simulink model "hcc_sm_v6_circuit"  (R2024b)
settings: Solver=VariableStepAuto  StartTime=0.0  StopTime=0.2  FixedStep=1e-7  RelTol=1e-3
libraries: spsSeriesRLCBranchLib x530, spsGtoLib x144, spsDiodeLib x78, spsCurrentMeasurementLib x6, spsVoltageMeasurementLib x6, spsGroundLib x3, spsDCVoltageSourceLib x1, spsThreePhaseProgrammableVoltageSourceLib x1, spsThreePhaseTransformerTwoWindingsLib x1, spsThreePhaseSourceLib x1, spspowerguiLib x1
(part 1 of 3)
settings Model: Creator=56305  LastModifiedBy=wei13
settings SolverCC: EnableFixedStepZeroCrossing=on
settings OptimizationCC: ReuseModelBlockBuffer=off
settings RTWCC: GPUComputeCapability=3.5

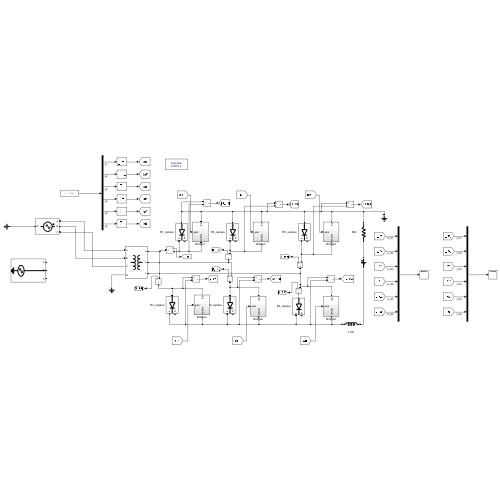
[thumbnail: Simulink's stored preview of the top-level diagram]
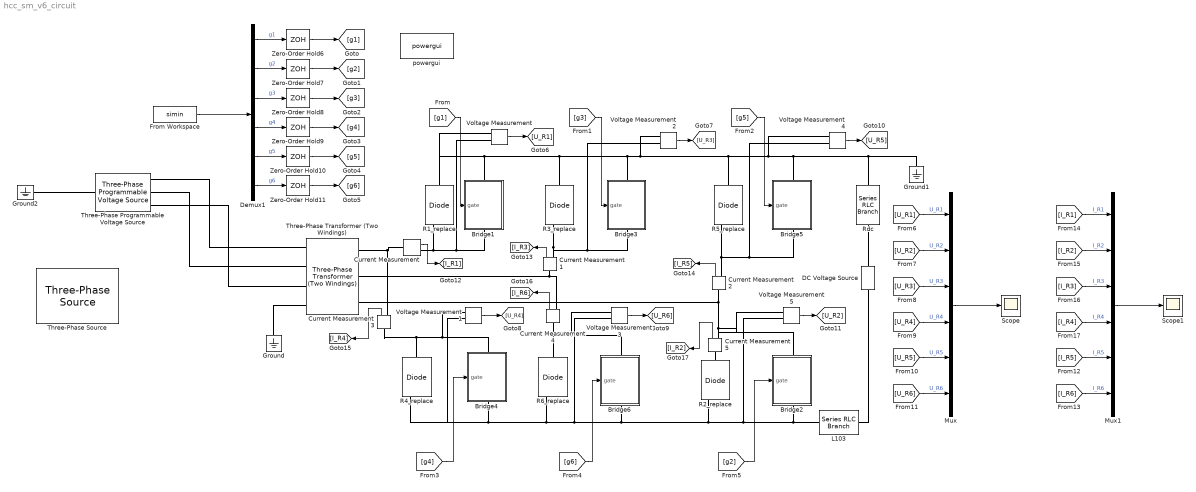
== system hcc_sm_v6_circuit ==
  Bridge1 : Subsystem
      settings: PortSchema="{\"entries\":[{\"content\":{\"sides\":[{\"content\":{\"connectorIds\":[\"In1\"]},\"type\":\"ConnectorPlacement.EquallySpacedRectSide\",\"uuid\":\"41aa3e2a-70f0-4b77-aa16-68e99ec54bcf\"},{\"content\":{\"side\":\"RIGHT\"},\"type\":\"ConnectorPlacement.EquallySpacedRectSide\",\"uuid\":\"96eb3ac2-20ab-4313-b955-709dae12ba5a\"},{\"content\":{\"connectorIds\":[\"LConn1\"],\"side\":\"TOP\"},\"type\":\"ConnectorPlacement.EquallySpacedRectSide\",\"uuid\":\"75cf1ed1-d1d6-43fb-a0f7-eae0627f950f\"},{\"content\":{\"connectorIds\":[\"RConn1\"],\"side\":\"BOTTOM\"},\"type\":\"ConnectorPlacement.EquallySpacedRectSide\",\"uuid\":\"e3d24c16-695e-4958-a9e5-c1041aebacaf\"}]},\"type\":\"ConnectorPlacement.EquallySpacedConnector\",\"uuid\":\"cea135f8-b684-4f22-bc6f-773380cf8880\"}],\"packageUris\":[\"http://schema.mathworks.com/mf0/Connector/R2020b\"],\"version\":\"1.0\"}"
  Bridge2 : Subsystem
      settings: PortSchema="{\"entries\":[{\"content\":{\"sides\":[{\"content\":{\"connectorIds\":[\"In1\"]},\"type\":\"ConnectorPlacement.EquallySpacedRectSide\",\"uuid\":\"41aa3e2a-70f0-4b77-aa16-68e99ec54bcf\"},{\"content\":{\"side\":\"RIGHT\"},\"type\":\"ConnectorPlacement.EquallySpacedRectSide\",\"uuid\":\"96eb3ac2-20ab-4313-b955-709dae12ba5a\"},{\"content\":{\"connectorIds\":[\"LConn1\"],\"side\":\"TOP\"},\"type\":\"ConnectorPlacement.EquallySpacedRectSide\",\"uuid\":\"75cf1ed1-d1d6-43fb-a0f7-eae0627f950f\"},{\"content\":{\"connectorIds\":[\"RConn1\"],\"side\":\"BOTTOM\"},\"type\":\"ConnectorPlacement.EquallySpacedRectSide\",\"uuid\":\"e3d24c16-695e-4958-a9e5-c1041aebacaf\"}]},\"type\":\"ConnectorPlacement.EquallySpacedConnector\",\"uuid\":\"cea135f8-b684-4f22-bc6f-773380cf8880\"}],\"packageUris\":[\"http://schema.mathworks.com/mf0/Connector/R2020b\"],\"version\":\"1.0\"}"
  Bridge3 : Subsystem
      settings: PortSchema="{\"entries\":[{\"content\":{\"sides\":[{\"content\":{\"connectorIds\":[\"In1\"]},\"type\":\"ConnectorPlacement.EquallySpacedRectSide\",\"uuid\":\"41aa3e2a-70f0-4b77-aa16-68e99ec54bcf\"},{\"content\":{\"side\":\"RIGHT\"},\"type\":\"ConnectorPlacement.EquallySpacedRectSide\",\"uuid\":\"96eb3ac2-20ab-4313-b955-709dae12ba5a\"},{\"content\":{\"connectorIds\":[\"LConn1\"],\"side\":\"TOP\"},\"type\":\"ConnectorPlacement.EquallySpacedRectSide\",\"uuid\":\"75cf1ed1-d1d6-43fb-a0f7-eae0627f950f\"},{\"content\":{\"connectorIds\":[\"RConn1\"],\"side\":\"BOTTOM\"},\"type\":\"ConnectorPlacement.EquallySpacedRectSide\",\"uuid\":\"e3d24c16-695e-4958-a9e5-c1041aebacaf\"}]},\"type\":\"ConnectorPlacement.EquallySpacedConnector\",\"uuid\":\"cea135f8-b684-4f22-bc6f-773380cf8880\"}],\"packageUris\":[\"http://schema.mathworks.com/mf0/Connector/R2020b\"],\"version\":\"1.0\"}"
  Bridge4 : Subsystem
      settings: PortSchema="{\"entries\":[{\"content\":{\"sides\":[{\"content\":{\"connectorIds\":[\"In1\"]},\"type\":\"ConnectorPlacement.EquallySpacedRectSide\",\"uuid\":\"41aa3e2a-70f0-4b77-aa16-68e99ec54bcf\"},{\"content\":{\"side\":\"RIGHT\"},\"type\":\"ConnectorPlacement.EquallySpacedRectSide\",\"uuid\":\"96eb3ac2-20ab-4313-b955-709dae12ba5a\"},{\"content\":{\"connectorIds\":[\"LConn1\"],\"side\":\"TOP\"},\"type\":\"ConnectorPlacement.EquallySpacedRectSide\",\"uuid\":\"75cf1ed1-d1d6-43fb-a0f7-eae0627f950f\"},{\"content\":{\"connectorIds\":[\"RConn1\"],\"side\":\"BOTTOM\"},\"type\":\"ConnectorPlacement.EquallySpacedRectSide\",\"uuid\":\"e3d24c16-695e-4958-a9e5-c1041aebacaf\"}]},\"type\":\"ConnectorPlacement.EquallySpacedConnector\",\"uuid\":\"cea135f8-b684-4f22-bc6f-773380cf8880\"}],\"packageUris\":[\"http://schema.mathworks.com/mf0/Connector/R2020b\"],\"version\":\"1.0\"}"
  Bridge5 : Subsystem
      settings: PortSchema="{\"entries\":[{\"content\":{\"sides\":[{\"content\":{\"connectorIds\":[\"In1\"]},\"type\":\"ConnectorPlacement.EquallySpacedRectSide\",\"uuid\":\"41aa3e2a-70f0-4b77-aa16-68e99ec54bcf\"},{\"content\":{\"side\":\"RIGHT\"},\"type\":\"ConnectorPlacement.EquallySpacedRectSide\",\"uuid\":\"96eb3ac2-20ab-4313-b955-709dae12ba5a\"},{\"content\":{\"connectorIds\":[\"LConn1\"],\"side\":\"TOP\"},\"type\":\"ConnectorPlacement.EquallySpacedRectSide\",\"uuid\":\"75cf1ed1-d1d6-43fb-a0f7-eae0627f950f\"},{\"content\":{\"connectorIds\":[\"RConn1\"],\"side\":\"BOTTOM\"},\"type\":\"ConnectorPlacement.EquallySpacedRectSide\",\"uuid\":\"e3d24c16-695e-4958-a9e5-c1041aebacaf\"}]},\"type\":\"ConnectorPlacement.EquallySpacedConnector\",\"uuid\":\"cea135f8-b684-4f22-bc6f-773380cf8880\"}],\"packageUris\":[\"http://schema.mathworks.com/mf0/Connector/R2020b\"],\"version\":\"1.0\"}"
  Bridge6 : Subsystem
      settings: PortSchema="{\"entries\":[{\"content\":{\"sides\":[{\"content\":{\"connectorIds\":[\"In1\"]},\"type\":\"ConnectorPlacement.EquallySpacedRectSide\",\"uuid\":\"41aa3e2a-70f0-4b77-aa16-68e99ec54bcf\"},{\"content\":{\"side\":\"RIGHT\"},\"type\":\"ConnectorPlacement.EquallySpacedRectSide\",\"uuid\":\"96eb3ac2-20ab-4313-b955-709dae12ba5a\"},{\"content\":{\"connectorIds\":[\"LConn1\"],\"side\":\"TOP\"},\"type\":\"ConnectorPlacement.EquallySpacedRectSide\",\"uuid\":\"75cf1ed1-d1d6-43fb-a0f7-eae0627f950f\"},{\"content\":{\"connectorIds\":[\"RConn1\"],\"side\":\"BOTTOM\"},\"type\":\"ConnectorPlacement.EquallySpacedRectSide\",\"uuid\":\"e3d24c16-695e-4958-a9e5-c1041aebacaf\"}]},\"type\":\"ConnectorPlacement.EquallySpacedConnector\",\"uuid\":\"cea135f8-b684-4f22-bc6f-773380cf8880\"}],\"packageUris\":[\"http://schema.mathworks.com/mf0/Connector/R2020b\"],\"version\":\"1.0\"}"
  Current Measurement{,1..5} (6 alike) : spsCurrentMeasurementLib/Current Measurement  PhasorSimulation=off  OutputType=Complex  PSBequivalent=0
  DC Voltage Source : spsDCVoltageSourceLib/DC Voltage Source  Amplitude=57000  Measurements=None
  Demux1 : Demux  Outputs=6
  From Workspace : FromWorkspace  VariableName=simin  SampleTime=0.0001  Interpolate=off  OutputAfterFinalValue=Holding final value
  Ground : spsGroundLib/Ground  LConnTagsString=a
  Ground1 : spsGroundLib/Ground  LConnTagsString=a
  Ground2 : spsGroundLib/Ground  LConnTagsString=a
  L103 : spsSeriesRLCBranchLib/Series RLC Branch  LConnTagsString=__new0  RConnTagsString=__new0  BranchType=L  Resistance=36  Inductance=120*1e-03  SetiL0=off  InitialCurrent=0  Capacitance=2.62e-06  Setx0=off  InitialVoltage=0  Measurements=None
  Mux : Mux  Inputs=6
  Mux1 : Mux  Inputs=6
  R1_replace : spsDiodeLib/Diode  Ron=3.2041  Lon=0  Vf=119772.7273  IC=0  UseSnubber=0  Rs=1e6  Cs=0  Measurements=on
  R2_replace : spsDiodeLib/Diode  Ron=3.2041  Lon=0  Vf=119772.7273  IC=0  UseSnubber=0  Rs=1e6  Cs=0  Measurements=on
  R3_replace : spsDiodeLib/Diode  Ron=3.2041  Lon=0  Vf=119772.7273  IC=0  UseSnubber=0  Rs=1e6  Cs=0  Measurements=on
  R4_replace : spsDiodeLib/Diode  Ron=3.2041  Lon=0  Vf=119772.7273  IC=0  UseSnubber=0  Rs=1e6  Cs=0  Measurements=on
  R5_replace : spsDiodeLib/Diode  Ron=3.2041  Lon=0  Vf=119772.7273  IC=0  UseSnubber=0  Rs=1e6  Cs=0  Measurements=on
  R6_replace : spsDiodeLib/Diode  Ron=3.2041  Lon=0  Vf=119772.7273  IC=0  UseSnubber=0  Rs=1e6  Cs=0  Measurements=on
  Rdc : spsSeriesRLCBranchLib/Series RLC Branch  LConnTagsString=__new0  RConnTagsString=__new0  BranchType=R  Resistance=1  Inductance=120e-03  SetiL0=off  InitialCurrent=0  Capacitance=2.62e-06  Setx0=off  InitialVoltage=0  Measurements=None
  Scope : Scope
  Scope1 : Scope
  Three-Phase Programmable Voltage Source : spsThreePhaseProgrammableVoltageSourceLib/Three-Phase Programmable Voltage Source  PositiveSequence="[345e3  0 50]"  VariationEntity=Amplitude  VariationType=Table of time-amplitude pairs  VariationTypeAlt=Step  VariationStep=0.5  VariationRate=1000  VariationMagnitude=0.3  VariationFrequency=2  VariationTiming=[0 1]  VariationPhaseA=off  Amplitudes=[0.000000 0.002000 0.004000 0.006000 0.008000 0.010000 0.012000 0.014000 0.016000 0.018000 0.020000 0.022000 0.024000 0.026000 0.028000 0.030000 0.032000 0.034000 0.036000 0.038000 0.040000 0.042000 0.044000 0.046000 0.048000 0.050000 0.052000 0.054000 0.056000 0.058000 0.060000 0.062000 0.064000 0.066000 0.068000 0.070000 0.072000 0.074000 0.076000 0.078000 0.080000 0.082000 0.084000 0.086000 0.088000 0.090000 0.092000 0.094000 0.096000 0.098000 0.100000 0.102000 0.104000 0.106000 0.108000 0.110000 0.112000 0.114000 0.116000 0.118000 0.120000 0.122000 0.124000 0.126000 0.128000 0.130000 0.132000 0.134000 0.136000 0.138000 0.140000 0.142000 0.144000 0.146000 0.148000 0.150000 0.152000 0.154000 0.156000 0.158000 0.160000 0.162000 0.164000 0.166000 0.168000 0.170000 0.172000 0.174000 0.176000 0.178000 0.180000 0.182000 0.184000 0.186000 0.188000 0.190000 0.192000 0.194000 0.196000 0.198000 0.200000 0.202000 0.204000 0.206000 0.208000 0.210000 0.212000 0.214000 0.216000 0.218000 0.220000 0.222000 0.224000 0.226000 0.228000 0.230000 0.232000 0.234000 0.236000 0.238000 0.240000 0.242000 0.244000 0.246000 0.248000 0.250000 0.252000 0.254000 0.256000 0.258000 0.260000 0.262000 0.264000 0.266000 0.268000 0.270000 0.272000 0.274000 0.276000 0.278000 0.280000 0.282000 0.284000 0.286000 0.288000 0.290000 0.292000 0.294000 0.296000 0.298000 0.300000 0.302000 0.304000 0.306000 0.308000 0.310000 0.312000 0.314000 0.316000 0.318000 0.320000 0.322000 0.324000 0.326000 0.328000 0.330000 0.332000 0.334000 0.336000 0.338000 0.340000 0.342000 0.344000 0.346000 0.348000 0.350000 0.352000 0.354000 0.356000 0.358000 0.360000 0.362000 0.364000 0.366000 0.368000 0.370000 0.372000 0.374000 0.376000 0.378000 0.380000 0.382000 0.384000 0.386000 0.388000 0.390000 0.392000 0.394000 0.396000 0.398000 0.400000 0.402000 0.404000 0.406000 0.408000 0.410000 0.412000 0.414000 0.416000 0.418000 0.420000 0.422000 0.424000 0.426000 0.428000 0.430000 0.432000 0.434000 0.436000 0.438000 0.440000 0.442000 0.444000 0.446000 0.448000 0.450000 0.452000 0.454000 0.456000 0.458000 0.460000 0.462000 0.464000 0.466000 0.468000 0.470000 0.472000 0.474000 0.476000 0.478000 0.480000 0.482000 0.484000 0.486000 0.488000 0.490000 0.492000 0.494000 0.496000 0.498000 0.500000 0.502000 0.504000 0.506000 0.508000 0.510000 0.512000 0.514000 0.516000 0.518000 0.520000 0.522000 0.524000 0.526000 0.528000 0.530000 0.532000 0.534000 0.536000 0.538000 0.540000 0.542000 0.544000 0.546000 0.548000 0.550000 0.552000 0.554000 0.556000 0.558000 0.560000 0.562000 0.564000 0.566000 0.568000 0.570000 0.572000 0.574000 0.576000 0.578000 0.580000 0.582000 0.584000 0.586000 0.588000 0.590000 0.592000 0.594000 0.596000 0.598000 0.600000 0.602000 0.604000 0.606000 0.608000 0.610000 0.612000 0.614000 0.616000 0.618000 0.620000 0.622000 0.624000 0.626000 0.628000 0.630000 0.632000 0.634000 0.636000 0.638000 0.640000 0.642000 0.644000 0.646000 0.648000 0.650000 0.652000 0.654000 0.656000 0.658000 0.660000 0.662000 0.664000 0.666000 0.668000 0.670000 0.672000 0.674000 0.676000 0.678000 0.680000 0.682000 0.684000 0.686000 0.688000 0.690000 0.692000 0.694000 0.696000 0.698000 0.700000 0.702000 0.704000 0.706000 0.708000 0.710000 0.712000 0.714000 0.716000 0.718000 0.720000 0.722000 0.724000 0.726000 0.728000 0.730000 0.732000 0.734000 0.736000 0.738000 0.740000 0.742000 0.744000 0.746000 0.748000 0.750000 0.752000 0.754000 0.756000 0.758000 0.760000 0.762000 0.764000 0.766000 0.768000 0.770000 0.772000 0.774000 0.776000 0.778000 0.780000 0.782000 0.784000 0.786000 0.788000 0.790000 0.792000 0.794000 0.796000 0.798000 0.800000 0.802000 0.804000 0.806000 0.808000 0.810000 0.812000 0.814000 0.816000 0.818000 0.820000 0.822000 0.824000 0.826000 0.828000 0.830000 0.832000 0.834000 0.836000 0.838000 0.840000 0.842000 0.844000 0.846000 0.848000 0.850000 0.852000 0.854000 0.856000 0.858000 0.860000 0.862000 0.864000 0.866000 0.868000 0.870000 0.872000 0.874000 0.876000 0.878000 0.880000 0.882000 0.884000 0.886000 ...(+513 chars) ]  TimeValues=[0.000000 0.000100 0.000200 0.000300 0.000400 0.000500 0.000600 0.000700 0.000800 0.000900 0.001000 0.001100 0.001200 0.001300 0.001400 0.001500 0.001600 0.001700 0.001800 0.001900 0.002000 0.002100 0.002200 0.002300 0.002400 0.002500 0.002600 0.002700 0.002800 0.002900 0.003000 0.003100 0.003200 0.003300 0.003400 0.003500 0.003600 0.003700 0.003800 0.003900 0.004000 0.004100 0.004200 0.004300 0.004400 0.004500 0.004600 0.004700 0.004800 0.004900 0.005000 0.005100 0.005200 0.005300 0.005400 0.005500 0.005600 0.005700 0.005800 0.005900 0.006000 0.006100 0.006200 0.006300 0.006400 0.006500 0.006600 0.006700 0.006800 0.006900 0.007000 0.007100 0.007200 0.007300 0.007400 0.007500 0.007600 0.007700 0.007800 0.007900 0.008000 0.008100 0.008200 0.008300 0.008400 0.008500 0.008600 0.008700 0.008800 0.008900 0.009000 0.009100 0.009200 0.009300 0.009400 0.009500 0.009600 0.009700 0.009800 0.009900 0.010000 0.010100 0.010200 0.010300 0.010400 0.010500 0.010600 0.010700 0.010800 0.010900 0.011000 0.011100 0.011200 0.011300 0.011400 0.011500 0.011600 0.011700 0.011800 0.011900 0.012000 0.012100 0.012200 0.012300 0.012400 0.012500 0.012600 0.012700 0.012800 0.012900 0.013000 0.013100 0.013200 0.013300 0.013400 0.013500 0.013600 0.013700 0.013800 0.013900 0.014000 0.014100 0.014200 0.014300 0.014400 0.014500 0.014600 0.014700 0.014800 0.014900 0.015000 0.015100 0.015200 0.015300 0.015400 0.015500 0.015600 0.015700 0.015800 0.015900 0.016000 0.016100 0.016200 0.016300 0.016400 0.016500 0.016600 0.016700 0.016800 0.016900 0.017000 0.017100 0.017200 0.017300 0.017400 0.017500 0.017600 0.017700 0.017800 0.017900 0.018000 0.018100 0.018200 0.018300 0.018400 0.018500 0.018600 0.018700 0.018800 0.018900 0.019000 0.019100 0.019200 0.019300 0.019400 0.019500 0.019600 0.019700 0.019800 0.019900 0.020000 0.020100 0.020200 0.020300 0.020400 0.020500 0.020600 0.020700 0.020800 0.020900 0.021000 0.021100 0.021200 0.021300 0.021400 0.021500 0.021600 0.021700 0.021800 0.021900 0.022000 0.022100 0.022200 0.022300 0.022400 0.022500 0.022600 0.022700 0.022800 0.022900 0.023000 0.023100 0.023200 0.023300 0.023400 0.023500 0.023600 0.023700 0.023800 0.023900 0.024000 0.024100 0.024200 0.024300 0.024400 0.024500 0.024600 0.024700 0.024800 0.024900 0.025000 0.025100 0.025200 0.025300 0.025400 0.025500 0.025600 0.025700 0.025800 0.025900 0.026000 0.026100 0.026200 0.026300 0.026400 0.026500 0.026600 0.026700 0.026800 0.026900 0.027000 0.027100 0.027200 0.027300 0.027400 0.027500 0.027600 0.027700 0.027800 0.027900 0.028000 0.028100 0.028200 0.028300 0.028400 0.028500 0.028600 0.028700 0.028800 0.028900 0.029000 0.029100 0.029200 0.029300 0.029400 0.029500 0.029600 0.029700 0.029800 0.029900 0.030000 0.030100 0.030200 0.030300 0.030400 0.030500 0.030600 0.030700 0.030800 0.030900 0.031000 0.031100 0.031200 0.031300 0.031400 0.031500 0.031600 0.031700 0.031800 0.031900 0.032000 0.032100 0.032200 0.032300 0.032400 0.032500 0.032600 0.032700 0.032800 0.032900 0.033000 0.033100 0.033200 0.033300 0.033400 0.033500 0.033600 0.033700 0.033800 0.033900 0.034000 0.034100 0.034200 0.034300 0.034400 0.034500 0.034600 0.034700 0.034800 0.034900 0.035000 0.035100 0.035200 0.035300 0.035400 0.035500 0.035600 0.035700 0.035800 0.035900 0.036000 0.036100 0.036200 0.036300 0.036400 0.036500 0.036600 0.036700 0.036800 0.036900 0.037000 0.037100 0.037200 0.037300 0.037400 0.037500 0.037600 0.037700 0.037800 0.037900 0.038000 0.038100 0.038200 0.038300 0.038400 0.038500 0.038600 0.038700 0.038800 0.038900 0.039000 0.039100 0.039200 0.039300 0.039400 0.039500 0.039600 0.039700 0.039800 0.039900 0.040000 0.040100 0.040200 0.040300 0.040400 0.040500 0.040600 0.040700 0.040800 0.040900 0.041000 0.041100 0.041200 0.041300 0.041400 0.041500 0.041600 0.041700 0.041800 0.041900 0.042000 0.042100 0.042200 0.042300 0.042400 0.042500 0.042600 0.042700 0.042800 0.042900 0.043000 0.043100 0.043200 0.043300 0.043400 0.043500 0.043600 0.043700 0.043800 0.043900 0.044000 0.044100 0.044200 0.044300 ...(+513 chars) ]  HarmonicGeneration=off  HarmonicA=[3 0.2 -25 0]  HarmonicB=[2 0.15 35 2]  Timing="[0.05  3]"  BusType=swing  Pref=0  Qref=0  Qmin=-inf  Qmax=inf
  Three-Phase Transformer (Two Windings) : spsThreePhaseTransformerTwoWindingsLib/Three-Phase Transformer (Two Windings)  Winding1Connection=Yn  Winding2Connection=Y  CoreType=Three single-phase transformers  SetSaturation=off  Hysteresis=off  DataFile='hysteresis'  SetInitialFlux=off  Measurements=None  UNITS=pu  NominalPower=[ 215.4e6 , 50 ]  Winding1=[ 345e3 , 0.002 , 0.08 ]  Winding2=[ 50.8e3 , 0.002 , 0.08 ]  Rm=500  Lm=500  L0=0.5  Saturation=[ 0,0 ; 0.0024,1.2 ; 1.0,1.52 ]  InitialFluxes=[ 0.8 , -0.8 , 0.7 ]  BreakLoop=off  DiscreteSolver=Trapezoidal iterative  DataType=off  TransfoNumber=1
  Three-Phase Source : spsThreePhaseSourceLib/Three-Phase Source  InternalConnection=Yg  VoltagePhases=off  Voltage=345e3  PhaseAngle=0  Voltage_phases=[25e3 25e3 25e3]/sqrt(3)  PhaseAngles_phases=[0 -120 +120]  Frequency=50  NonIdealSource=off  SpecifyImpedance=off  Resistance=0  Inductance=0  ShortCircuitLevel=100e6  BaseVoltage=25e3  XRratio=7  BusType=swing  Pref=10e3  Qref=0  Prefabc=[10e3, 10e3, 10e3]  Qrefabc=[0, 0, 0]  Qmin=-inf  Qmax=inf
  Voltage Measurement{,1..5} (6 alike) : spsVoltageMeasurementLib/Voltage Measurement  PhasorSimulation=off  OutputType=Complex  PSBequivalent=0
  Zero-Order Hold{6..11} (6 alike) : ZeroOrderHold  SampleTime=1e-4
  powergui : spspowerguiLib/powergui  Priority=1  SimulationMode=Discrete  SampleTime=1e-4  frequency=60  Iterations=50  frequencyindice=50  Pbase=100e6  ErrMax=1e-4  UnitsV=kV  UnitsW=MW  buscounter=0  FunctionMessages=off  echomessages=off  EnableUseOfTLC=off  CurrentSourceSwitches=off  DisableSnubberDevices=off  DisableRonSwitches=off  DisableVfSwitches=off  DisplayEquations=off  AutomaticDiscreteSolvers=off  SolverType=Tustin/Backward Euler (TBE)  Interpol=off  ExternalGateDelay=off  methode=off  Ts=100  x0status=blocks  SPID=on  SwTol=0  HookPort=off  NonlinearTolerance=1e-4  nMaxIteration=1000  ContinueOnMaxIteration=off  RestoreLinks=warning  ResistiveCurrentMeasurement=off  Frange=[0:2:500]  Ylog=off  Xlog=on  ShowGrid=off  save=off  variable=ZData  structure=0  ZoomFFT=off  StartTime=0.0  cycles=1  DisplayStyle=1  fundamental=60  FreqAxis=off  MaxFrequency=1000  frequencyindicesteady=1  RmsSteady=1  display=off
  wires:
  From Workspace/1 -> Demux1/1
  [g1] -> Bridge1/1(gate)
  [g3] -> Bridge3/1(gate)
  [g5] -> Bridge5/1(gate)
  [g4] -> Bridge4/1(gate)
  [g6] -> Bridge6/1(gate)
  [g2] -> Bridge2/1(gate)
  Voltage Measurement/1 -> [U_R1]
  Voltage Measurement2/1 -> [U_R3]
  Voltage Measurement1/1 -> [U_R4]
  Voltage Measurement3/1 -> [U_R6]
  Voltage Measurement4/1 -> [U_R5]
  Voltage Measurement5/1 -> [U_R2]
  [U_R1] -> Mux/1  "U_R1"
  [U_R2] -> Mux/2  "U_R2"
  [U_R3] -> Mux/3  "U_R3"
  [U_R4] -> Mux/4  "U_R4"
  [U_R5] -> Mux/5  "U_R5"
  [U_R6] -> Mux/6  "U_R6"
  Mux/1 -> Scope/1
  Demux1/2 -> Zero-Order Hold7/1  "g2"
  Demux1/1 -> Zero-Order Hold6/1  "g1"
  Demux1/3 -> Zero-Order Hold8/1  "g3"
  Demux1/4 -> Zero-Order Hold9/1  "g4"
  Demux1/5 -> Zero-Order Hold10/1  "g5"
  Demux1/6 -> Zero-Order Hold11/1  "g6"
  Zero-Order Hold6/1 -> [g1]
  Zero-Order Hold7/1 -> [g2]
  Zero-Order Hold8/1 -> [g3]
  Zero-Order Hold9/1 -> [g4]
  Zero-Order Hold10/1 -> [g5]
  Zero-Order Hold11/1 -> [g6]
  Current Measurement/1 -> [I_R1]
  Current Measurement1/1 -> [I_R3]
  Current Measurement2/1 -> [I_R5]
  Current Measurement3/1 -> [I_R4]
  Current Measurement4/1 -> [I_R6]
  Current Measurement5/1 -> [I_R2]
  Mux1/1 -> Scope1/1
  [I_R4] -> Mux1/4  "I_R4"
  [I_R5] -> Mux1/5  "I_R5"
  [I_R3] -> Mux1/3  "I_R3"
  [I_R2] -> Mux1/2  "I_R2"
  [I_R1] -> Mux1/1  "I_R1"
  [I_R6] -> Mux1/6  "I_R6"
  connections:
  Three-Phase Transformer (Two Windings)/LConn4 -- Ground/LConn1
  R4_replace/LConn1 -- Current Measurement3/LConn1 -- Bridge4/LConn1 -- Voltage Measurement1/LConn1
  R3_replace/RConn1 -- Bridge3/RConn1 -- Voltage Measurement2/LConn2 -- Current Measurement1/RConn1
  Three-Phase Transformer (Two Windings)/RConn3 -- Bridge2/LConn1 -- Voltage Measurement5/LConn1 -- Current Measurement5/RConn1 -- Current Measurement2/LConn1
  L103/LConn1 -- Bridge2/RConn1 -- Voltage Measurement5/LConn2 -- R2_replace/RConn1 -- Bridge6/RConn1 -- Voltage Measurement3/LConn2 -- R6_replace/RConn1 -- Bridge4/RConn1 -- Voltage Measurement1/LConn2 -- R4_replace/RConn1
  DC Voltage Source/RConn1 -- Rdc/RConn1
  Voltage Measurement/LConn1 -- R1_replace/LConn1 -- Bridge1/LConn1 -- R3_replace/LConn1 -- Bridge3/LConn1 -- Voltage Measurement2/LConn1 -- R5_replace/LConn1 -- Voltage Measurement4/LConn1 -- Bridge5/LConn1 -- Rdc/LConn1 -- Ground1/LConn1
  L103/RConn1 -- DC Voltage Source/LConn1
  Ground2/LConn1 -- Three-Phase Programmable Voltage Source/LConn1
  Three-Phase Transformer (Two Windings)/LConn3 -- Three-Phase Programmable Voltage Source/RConn3
  Three-Phase Programmable Voltage Source/RConn2 -- Three-Phase Transformer (Two Windings)/LConn2
  Three-Phase Transformer (Two Windings)/LConn1 -- Three-Phase Programmable Voltage Source/RConn1
  R1_replace/RConn1 -- Bridge1/RConn1 -- Voltage Measurement/LConn2 -- Current Measurement/RConn1
  Three-Phase Transformer (Two Windings)/RConn2 -- Current Measurement4/RConn1 -- Current Measurement1/LConn1
  Bridge5/RConn1 -- Voltage Measurement4/LConn2 -- Current Measurement2/RConn1 -- R5_replace/RConn1
  Three-Phase Transformer (Two Windings)/RConn1 -- Current Measurement3/RConn1 -- Current Measurement/LConn1
  R6_replace/LConn1 -- Current Measurement4/LConn1 -- Bridge6/LConn1 -- Voltage Measurement3/LConn1
  Current Measurement5/LConn1 -- R2_replace/LConn1

== system hcc_sm_v6_circuit/Bridge1 ==
  gate : Inport
  Segment1 : Subsystem
  Segment2 : Subsystem
  Segment3 : Subsystem
  Segment4 : Subsystem
  top : PMIOPort  Side=Left
  bottom : PMIOPort  Port=2  Side=Right
  wires:
  gate/1 -> Segment2/1(gate), Segment4/1(gate), Segment3/1(gate), Segment1/1(gate)
  connections:
  Segment2/LConn1 -- Segment1/RConn1
  Segment3/LConn1 -- Segment2/RConn1
  Segment4/LConn1 -- Segment3/RConn1
  Segment1/LConn1 -- top/RConn1
  Segment4/RConn1 -- bottom/RConn1

== system hcc_sm_v6_circuit/Bridge2 ==
  gate : Inport
  Segment1 : Subsystem
  Segment2 : Subsystem
  Segment3 : Subsystem
  Segment4 : Subsystem
  top : PMIOPort  Side=Left
  bottom : PMIOPort  Port=2  Side=Right
  wires:
  gate/1 -> Segment1/1(gate), Segment3/1(gate), Segment4/1(gate), Segment2/1(gate)
  connections:
  Segment4/RConn1 -- bottom/RConn1
  Segment1/LConn1 -- top/RConn1
  Segment4/LConn1 -- Segment3/RConn1
  Segment3/LConn1 -- Segment2/RConn1
  Segment2/LConn1 -- Segment1/RConn1

== system hcc_sm_v6_circuit/Bridge3 ==
  gate : Inport
  Segment1 : Subsystem
  Segment2 : Subsystem
  Segment3 : Subsystem
  Segment4 : Subsystem
  top : PMIOPort  Side=Left
  bottom : PMIOPort  Port=2  Side=Right
  wires:
  gate/1 -> Segment2/1(gate), Segment4/1(gate), Segment3/1(gate), Segment1/1(gate)
  connections:
  Segment2/LConn1 -- Segment1/RConn1
  Segment3/LConn1 -- Segment2/RConn1
  Segment4/LConn1 -- Segment3/RConn1
  Segment1/LConn1 -- top/RConn1
  Segment4/RConn1 -- bottom/RConn1

== system hcc_sm_v6_circuit/Bridge4 ==
  gate : Inport
  Segment1 : Subsystem
  Segment2 : Subsystem
  Segment3 : Subsystem
  Segment4 : Subsystem
  top : PMIOPort  Side=Left
  bottom : PMIOPort  Port=2  Side=Right
  wires:
  gate/1 -> Segment1/1(gate), Segment3/1(gate), Segment4/1(gate), Segment2/1(gate)
  connections:
  Segment4/RConn1 -- bottom/RConn1
  Segment1/LConn1 -- top/RConn1
  Segment4/LConn1 -- Segment3/RConn1
  Segment3/LConn1 -- Segment2/RConn1
  Segment2/LConn1 -- Segment1/RConn1

== system hcc_sm_v6_circuit/Bridge5 ==
  gate : Inport
  Segment1 : Subsystem
  Segment2 : Subsystem
  Segment3 : Subsystem
  Segment4 : Subsystem
  top : PMIOPort  Side=Left
  bottom : PMIOPort  Port=2  Side=Right
  wires:
  gate/1 -> Segment2/1(gate), Segment4/1(gate), Segment3/1(gate), Segment1/1(gate)
  connections:
  Segment2/LConn1 -- Segment1/RConn1
  Segment3/LConn1 -- Segment2/RConn1
  Segment4/LConn1 -- Segment3/RConn1
  Segment1/LConn1 -- top/RConn1
  Segment4/RConn1 -- bottom/RConn1

== system hcc_sm_v6_circuit/Bridge6 ==
  gate : Inport
  Segment1 : Subsystem
  Segment2 : Subsystem
  Segment3 : Subsystem
  Segment4 : Subsystem
  top : PMIOPort  Side=Left
  bottom : PMIOPort  Port=2  Side=Right
  wires:
  gate/1 -> Segment1/1(gate), Segment3/1(gate), Segment4/1(gate), Segment2/1(gate)
  connections:
  Segment4/RConn1 -- bottom/RConn1
  Segment1/LConn1 -- top/RConn1
  Segment4/LConn1 -- Segment3/RConn1
  Segment3/LConn1 -- Segment2/RConn1
  Segment2/LConn1 -- Segment1/RConn1

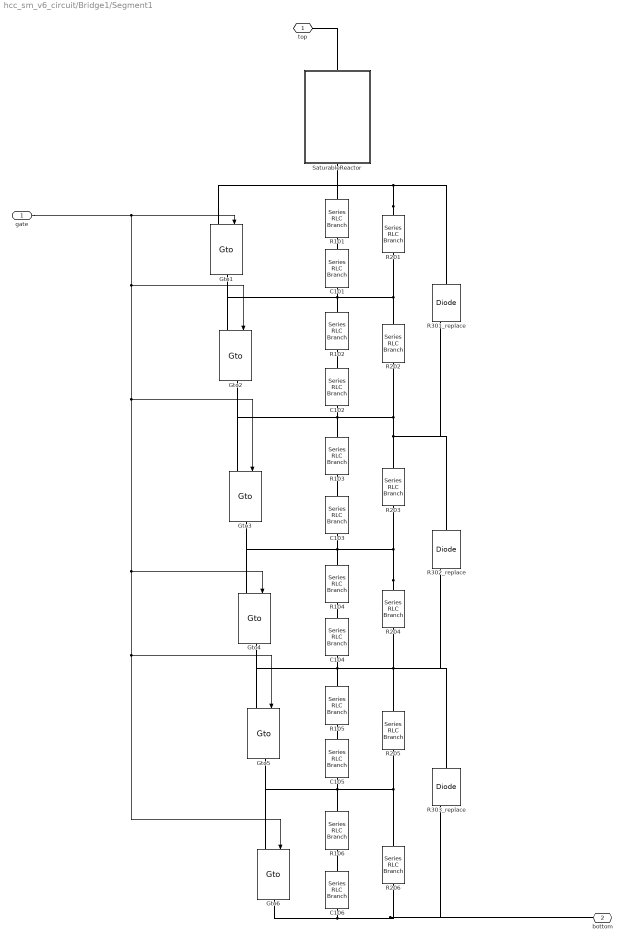
== system hcc_sm_v6_circuit/Bridge1/Segment1 ==
  gate : Inport
  C{101..106} (6 alike) : spsSeriesRLCBranchLib/Series RLC Branch  LConnTagsString=__new0  RConnTagsString=__new0  BranchType=C  Resistance=350  Inductance=107.42e-03  SetiL0=off  InitialCurrent=0  Capacitance=2.2*1e-6  Setx0=off  InitialVoltage=0  Measurements=None
  Gto{1..6} (6 alike) : spsGtoLib/Gto  Ron=0.226e-3  Lon=0  Vf=1.2  Tf=10e-6  Tt=20e-6  IC=0  Rs=161.25e3  Cs=0  Measurements=off
  R{101..106} (6 alike) : spsSeriesRLCBranchLib/Series RLC Branch  LConnTagsString=__new0  RConnTagsString=__new0  BranchType=R  Resistance=36  Inductance=107.42e-03  SetiL0=off  InitialCurrent=0  Capacitance=2.62e-06  Setx0=off  InitialVoltage=0  Measurements=None
  R{201..206} (6 alike) : spsSeriesRLCBranchLib/Series RLC Branch  LConnTagsString=__new0  RConnTagsString=__new0  BranchType=R  Resistance=88*1e3  Inductance=107.42e-03  SetiL0=off  InitialCurrent=0  Capacitance=2.62e-06  Setx0=off  InitialVoltage=0  Measurements=None
  R301_replace : spsDiodeLib/Diode  Ron=0.2624  Lon=0  Vf=11825.10104  IC=0  UseSnubber=0  Rs=1e6  Cs=0  Measurements=on
  R302_replace : spsDiodeLib/Diode  Ron=0.2624  Lon=0  Vf=11825.10104  IC=0  UseSnubber=0  Rs=1e6  Cs=0  Measurements=on
  R303_replace : spsDiodeLib/Diode  Ron=0.2624  Lon=0  Vf=11825.10104  IC=0  UseSnubber=0  Rs=1e6  Cs=0  Measurements=on
  SaturableReactor : Subsystem
  top : PMIOPort  Side=Left
  bottom : PMIOPort  Port=2  Side=Right
  wires:
  gate/1 -> Gto3/1, Gto4/1, Gto6/1, Gto5/1, Gto2/1, Gto1/1
  connections:
  R201/RConn1 -- Gto2/LConn1 -- Gto1/RConn1 -- C101/RConn1 -- R102/LConn1 -- R202/LConn1
  R204/LConn1 -- R203/RConn1 -- C103/RConn1 -- Gto4/LConn1 -- Gto3/RConn1 -- R104/LConn1
  R201/LConn1 -- R301_replace/LConn1 -- Gto1/LConn1 -- SaturableReactor/RConn1 -- R101/LConn1
  R205/RConn1 -- C105/RConn1 -- R106/LConn1 -- Gto6/LConn1 -- Gto5/RConn1 -- R206/LConn1
  R202/RConn1 -- C102/RConn1 -- Gto3/LConn1 -- Gto2/RConn1 -- R103/LConn1 -- R203/LConn1 -- R302_replace/LConn1 -- R301_replace/RConn1
  C106/RConn1 -- Gto6/RConn1 -- R206/RConn1 -- R303_replace/RConn1 -- bottom/RConn1
  SaturableReactor/LConn1 -- top/RConn1
  C101/LConn1 -- R101/RConn1
  C102/LConn1 -- R102/RConn1
  R103/RConn1 -- C103/LConn1
  R104/RConn1 -- C104/LConn1
  R105/RConn1 -- C105/LConn1
  R106/RConn1 -- C106/LConn1
  R105/LConn1 -- C104/RConn1 -- Gto5/LConn1 -- Gto4/RConn1 -- R303_replace/LConn1 -- R302_replace/RConn1 -- R205/LConn1 -- R204/RConn1

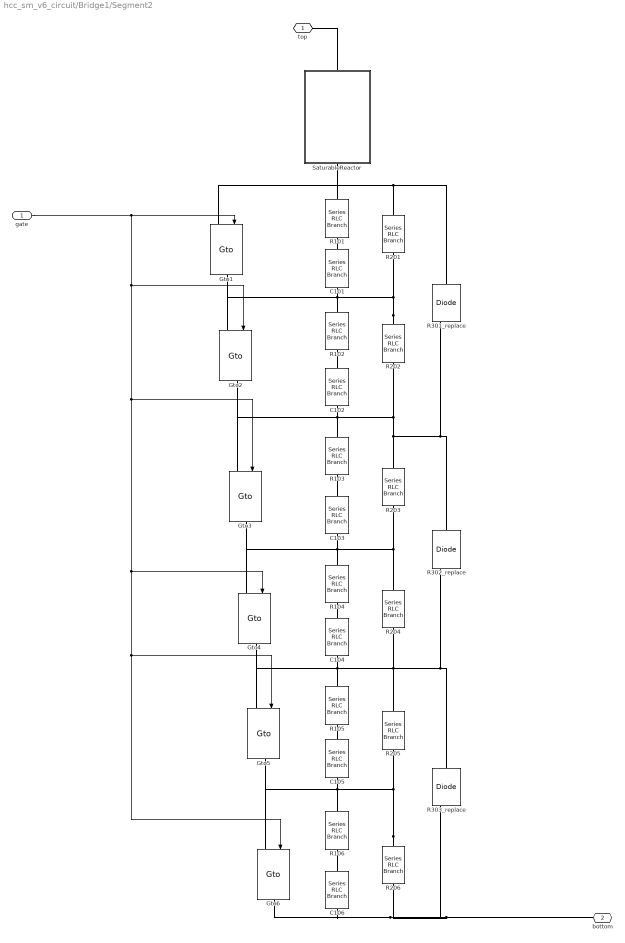
== system hcc_sm_v6_circuit/Bridge1/Segment2 ==
  gate : Inport
  C{101..106} (6 alike) : spsSeriesRLCBranchLib/Series RLC Branch  LConnTagsString=__new0  RConnTagsString=__new0  BranchType=C  Resistance=350  Inductance=107.42e-03  SetiL0=off  InitialCurrent=0  Capacitance=2.2*1e-6  Setx0=off  InitialVoltage=0  Measurements=None
  Gto{1..6} (6 alike) : spsGtoLib/Gto  Ron=0.226e-3  Lon=0  Vf=1.2  Tf=10e-6  Tt=20e-6  IC=0  Rs=161.25e3  Cs=0  Measurements=off
  R{101..106} (6 alike) : spsSeriesRLCBranchLib/Series RLC Branch  LConnTagsString=__new0  RConnTagsString=__new0  BranchType=R  Resistance=36  Inductance=107.42e-03  SetiL0=off  InitialCurrent=0  Capacitance=2.62e-06  Setx0=off  InitialVoltage=0  Measurements=None
  R{201..206} (6 alike) : spsSeriesRLCBranchLib/Series RLC Branch  LConnTagsString=__new0  RConnTagsString=__new0  BranchType=R  Resistance=88*1e3  Inductance=107.42e-03  SetiL0=off  InitialCurrent=0  Capacitance=2.62e-06  Setx0=off  InitialVoltage=0  Measurements=None
  R301_replace : spsDiodeLib/Diode  Ron=0.2624  Lon=0  Vf=11825.10104  IC=0  UseSnubber=0  Rs=1e6  Cs=0  Measurements=on
  R302_replace : spsDiodeLib/Diode  Ron=0.2624  Lon=0  Vf=11825.10104  IC=0  UseSnubber=0  Rs=1e6  Cs=0  Measurements=on
  R303_replace : spsDiodeLib/Diode  Ron=0.2624  Lon=0  Vf=11825.10104  IC=0  UseSnubber=0  Rs=1e6  Cs=0  Measurements=on
  SaturableReactor : Subsystem
  top : PMIOPort  Side=Left
  bottom : PMIOPort  Port=2  Side=Right
  wires:
  gate/1 -> Gto1/1, Gto2/1, Gto5/1, Gto6/1, Gto4/1, Gto3/1
  connections:
  R303_replace/LConn1 -- R204/RConn1 -- R205/LConn1 -- Gto4/RConn1 -- Gto5/LConn1 -- C104/RConn1 -- R105/LConn1 -- R302_replace/RConn1
  R106/RConn1 -- C106/LConn1
  R105/RConn1 -- C105/LConn1
  R104/RConn1 -- C104/LConn1
  R103/RConn1 -- C103/LConn1
  C102/LConn1 -- R102/RConn1
  C101/LConn1 -- R101/RConn1
  SaturableReactor/LConn1 -- top/RConn1
  R303_replace/RConn1 -- R206/RConn1 -- Gto6/RConn1 -- C106/RConn1 -- bottom/RConn1
  R302_replace/LConn1 -- R203/LConn1 -- R103/LConn1 -- Gto2/RConn1 -- Gto3/LConn1 -- C102/RConn1 -- R202/RConn1 -- R301_replace/RConn1
  R206/LConn1 -- Gto5/RConn1 -- Gto6/LConn1 -- R106/LConn1 -- C105/RConn1 -- R205/RConn1
  R301_replace/LConn1 -- R101/LConn1 -- SaturableReactor/RConn1 -- Gto1/LConn1 -- R201/LConn1
  R104/LConn1 -- Gto3/RConn1 -- Gto4/LConn1 -- C103/RConn1 -- R203/RConn1 -- R204/LConn1
  R202/LConn1 -- R102/LConn1 -- C101/RConn1 -- Gto1/RConn1 -- Gto2/LConn1 -- R201/RConn1

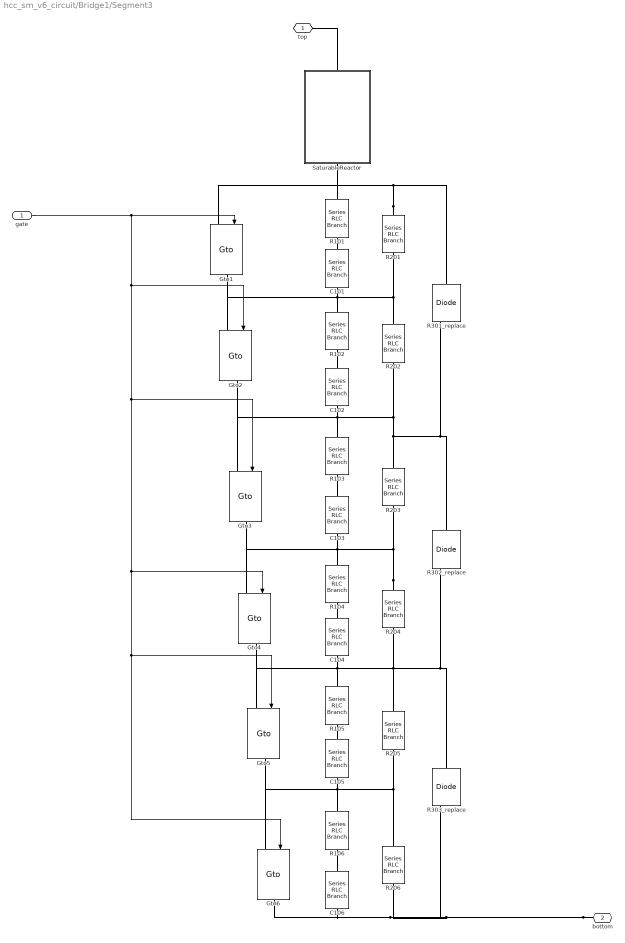
== system hcc_sm_v6_circuit/Bridge1/Segment3 ==
  gate : Inport
  C{101..106} (6 alike) : spsSeriesRLCBranchLib/Series RLC Branch  LConnTagsString=__new0  RConnTagsString=__new0  BranchType=C  Resistance=350  Inductance=107.42e-03  SetiL0=off  InitialCurrent=0  Capacitance=2.2*1e-6  Setx0=off  InitialVoltage=0  Measurements=None
  Gto{1..6} (6 alike) : spsGtoLib/Gto  Ron=0.226e-3  Lon=0  Vf=1.2  Tf=10e-6  Tt=20e-6  IC=0  Rs=161.25e3  Cs=0  Measurements=off
  R{101..106} (6 alike) : spsSeriesRLCBranchLib/Series RLC Branch  LConnTagsString=__new0  RConnTagsString=__new0  BranchType=R  Resistance=36  Inductance=107.42e-03  SetiL0=off  InitialCurrent=0  Capacitance=2.62e-06  Setx0=off  InitialVoltage=0  Measurements=None
  R{201..206} (6 alike) : spsSeriesRLCBranchLib/Series RLC Branch  LConnTagsString=__new0  RConnTagsString=__new0  BranchType=R  Resistance=88*1e3  Inductance=107.42e-03  SetiL0=off  InitialCurrent=0  Capacitance=2.62e-06  Setx0=off  InitialVoltage=0  Measurements=None
  R301_replace : spsDiodeLib/Diode  Ron=0.2624  Lon=0  Vf=11825.10104  IC=0  UseSnubber=0  Rs=1e6  Cs=0  Measurements=on
  R302_replace : spsDiodeLib/Diode  Ron=0.2624  Lon=0  Vf=11825.10104  IC=0  UseSnubber=0  Rs=1e6  Cs=0  Measurements=on
  R303_replace : spsDiodeLib/Diode  Ron=0.2624  Lon=0  Vf=11825.10104  IC=0  UseSnubber=0  Rs=1e6  Cs=0  Measurements=on
  SaturableReactor : Subsystem
  top : PMIOPort  Side=Left
  bottom : PMIOPort  Port=2  Side=Right
  wires:
  gate/1 -> Gto3/1, Gto4/1, Gto6/1, Gto5/1, Gto2/1, Gto1/1
  connections:
  R201/RConn1 -- Gto2/LConn1 -- Gto1/RConn1 -- C101/RConn1 -- R102/LConn1 -- R202/LConn1
  R204/LConn1 -- R203/RConn1 -- C103/RConn1 -- Gto4/LConn1 -- Gto3/RConn1 -- R104/LConn1
  R201/LConn1 -- Gto1/LConn1 -- SaturableReactor/RConn1 -- R101/LConn1 -- R301_replace/LConn1
  R205/RConn1 -- C105/RConn1 -- R106/LConn1 -- Gto6/LConn1 -- Gto5/RConn1 -- R206/LConn1
  R301_replace/RConn1 -- R202/RConn1 -- C102/RConn1 -- Gto3/LConn1 -- Gto2/RConn1 -- R103/LConn1 -- R203/LConn1 -- R302_replace/LConn1
  bottom/RConn1 -- C106/RConn1 -- Gto6/RConn1 -- R206/RConn1 -- R303_replace/RConn1
  SaturableReactor/LConn1 -- top/RConn1
  C101/LConn1 -- R101/RConn1
  C102/LConn1 -- R102/RConn1
  R103/RConn1 -- C103/LConn1
  R104/RConn1 -- C104/LConn1
  R105/RConn1 -- C105/LConn1
  R106/RConn1 -- C106/LConn1
  R302_replace/RConn1 -- R105/LConn1 -- C104/RConn1 -- Gto5/LConn1 -- Gto4/RConn1 -- R205/LConn1 -- R204/RConn1 -- R303_replace/LConn1

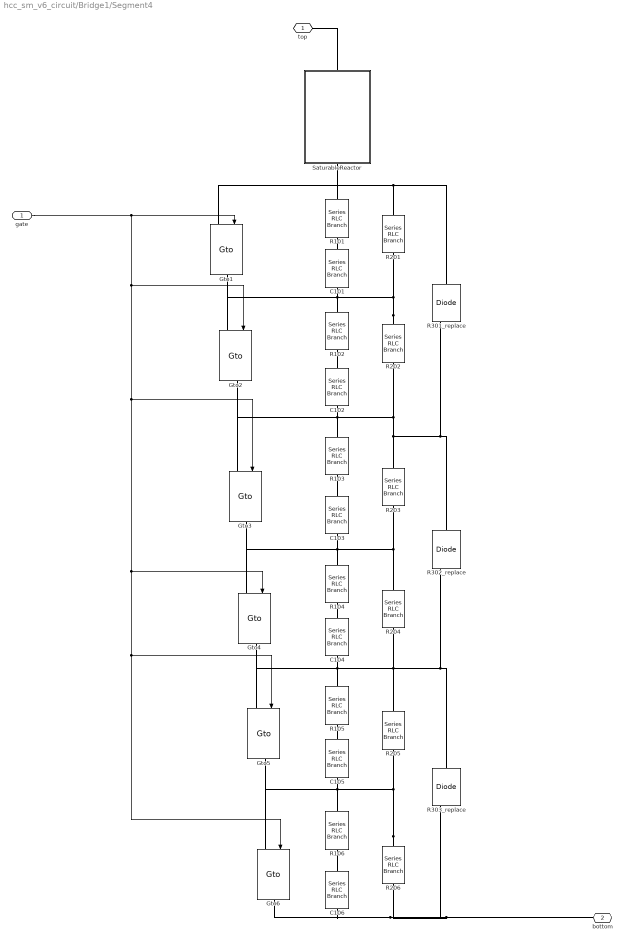
== system hcc_sm_v6_circuit/Bridge1/Segment4 ==
  gate : Inport
  C{101..106} (6 alike) : spsSeriesRLCBranchLib/Series RLC Branch  LConnTagsString=__new0  RConnTagsString=__new0  BranchType=C  Resistance=350  Inductance=107.42e-03  SetiL0=off  InitialCurrent=0  Capacitance=2.2*1e-6  Setx0=off  InitialVoltage=0  Measurements=None
  Gto{1..6} (6 alike) : spsGtoLib/Gto  Ron=0.226e-3  Lon=0  Vf=1.2  Tf=10e-6  Tt=20e-6  IC=0  Rs=161.25e3  Cs=0  Measurements=off
  R{101..106} (6 alike) : spsSeriesRLCBranchLib/Series RLC Branch  LConnTagsString=__new0  RConnTagsString=__new0  BranchType=R  Resistance=36  Inductance=107.42e-03  SetiL0=off  InitialCurrent=0  Capacitance=2.62e-06  Setx0=off  InitialVoltage=0  Measurements=None
  R{201..206} (6 alike) : spsSeriesRLCBranchLib/Series RLC Branch  LConnTagsString=__new0  RConnTagsString=__new0  BranchType=R  Resistance=88*1e3  Inductance=107.42e-03  SetiL0=off  InitialCurrent=0  Capacitance=2.62e-06  Setx0=off  InitialVoltage=0  Measurements=None
  R301_replace : spsDiodeLib/Diode  Ron=0.2624  Lon=0  Vf=11825.10104  IC=0  UseSnubber=0  Rs=1e6  Cs=0  Measurements=on
  R302_replace : spsDiodeLib/Diode  Ron=0.2624  Lon=0  Vf=11825.10104  IC=0  UseSnubber=0  Rs=1e6  Cs=0  Measurements=on
  R303_replace : spsDiodeLib/Diode  Ron=0.2624  Lon=0  Vf=11825.10104  IC=0  UseSnubber=0  Rs=1e6  Cs=0  Measurements=on
  SaturableReactor : Subsystem
  top : PMIOPort  Side=Left
  bottom : PMIOPort  Port=2  Side=Right
  wires:
  gate/1 -> Gto1/1, Gto2/1, Gto5/1, Gto6/1, Gto4/1, Gto3/1
  connections:
  R303_replace/LConn1 -- R204/RConn1 -- R205/LConn1 -- Gto4/RConn1 -- Gto5/LConn1 -- C104/RConn1 -- R105/LConn1 -- R302_replace/RConn1
  R106/RConn1 -- C106/LConn1
  R105/RConn1 -- C105/LConn1
  R104/RConn1 -- C104/LConn1
  R103/RConn1 -- C103/LConn1
  C102/LConn1 -- R102/RConn1
  C101/LConn1 -- R101/RConn1
  SaturableReactor/LConn1 -- top/RConn1
  R303_replace/RConn1 -- R206/RConn1 -- Gto6/RConn1 -- C106/RConn1 -- bottom/RConn1
  R302_replace/LConn1 -- R203/LConn1 -- R103/LConn1 -- Gto2/RConn1 -- Gto3/LConn1 -- C102/RConn1 -- R202/RConn1 -- R301_replace/RConn1
  R206/LConn1 -- Gto5/RConn1 -- Gto6/LConn1 -- R106/LConn1 -- C105/RConn1 -- R205/RConn1
  R301_replace/LConn1 -- R101/LConn1 -- SaturableReactor/RConn1 -- Gto1/LConn1 -- R201/LConn1
  R104/LConn1 -- Gto3/RConn1 -- Gto4/LConn1 -- C103/RConn1 -- R203/RConn1 -- R204/LConn1
  R202/LConn1 -- R102/LConn1 -- C101/RConn1 -- Gto1/RConn1 -- Gto2/LConn1 -- R201/RConn1

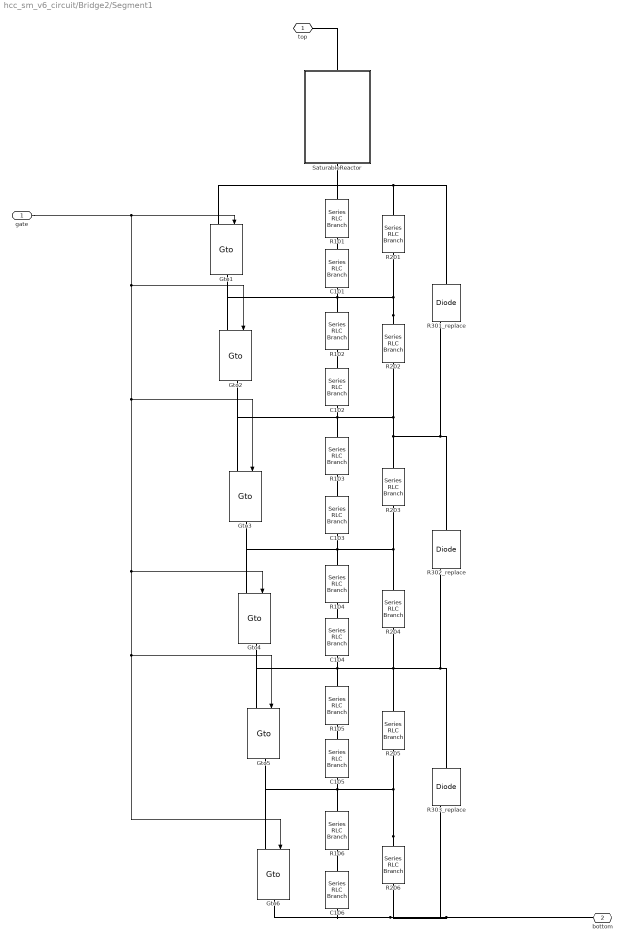
== system hcc_sm_v6_circuit/Bridge2/Segment1 ==
  gate : Inport
  C{101..106} (6 alike) : spsSeriesRLCBranchLib/Series RLC Branch  LConnTagsString=__new0  RConnTagsString=__new0  BranchType=C  Resistance=350  Inductance=107.42e-03  SetiL0=off  InitialCurrent=0  Capacitance=2.2*1e-6  Setx0=off  InitialVoltage=0  Measurements=None
  Gto{1..6} (6 alike) : spsGtoLib/Gto  Ron=0.226e-3  Lon=0  Vf=1.2  Tf=10e-6  Tt=20e-6  IC=0  Rs=161.25e3  Cs=0  Measurements=off
  R{101..106} (6 alike) : spsSeriesRLCBranchLib/Series RLC Branch  LConnTagsString=__new0  RConnTagsString=__new0  BranchType=R  Resistance=36  Inductance=107.42e-03  SetiL0=off  InitialCurrent=0  Capacitance=2.62e-06  Setx0=off  InitialVoltage=0  Measurements=None
  R{201..206} (6 alike) : spsSeriesRLCBranchLib/Series RLC Branch  LConnTagsString=__new0  RConnTagsString=__new0  BranchType=R  Resistance=88*1e3  Inductance=107.42e-03  SetiL0=off  InitialCurrent=0  Capacitance=2.62e-06  Setx0=off  InitialVoltage=0  Measurements=None
  R301_replace : spsDiodeLib/Diode  Ron=0.2624  Lon=0  Vf=11825.10104  IC=0  UseSnubber=0  Rs=1e6  Cs=0  Measurements=on
  R302_replace : spsDiodeLib/Diode  Ron=0.2624  Lon=0  Vf=11825.10104  IC=0  UseSnubber=0  Rs=1e6  Cs=0  Measurements=on
  R303_replace : spsDiodeLib/Diode  Ron=0.2624  Lon=0  Vf=11825.10104  IC=0  UseSnubber=0  Rs=1e6  Cs=0  Measurements=on
  SaturableReactor : Subsystem
  top : PMIOPort  Side=Left
  bottom : PMIOPort  Port=2  Side=Right
  wires:
  gate/1 -> Gto1/1, Gto2/1, Gto5/1, Gto6/1, Gto4/1, Gto3/1
  connections:
  R303_replace/LConn1 -- R204/RConn1 -- R205/LConn1 -- Gto4/RConn1 -- Gto5/LConn1 -- C104/RConn1 -- R105/LConn1 -- R302_replace/RConn1
  R106/RConn1 -- C106/LConn1
  R105/RConn1 -- C105/LConn1
  R104/RConn1 -- C104/LConn1
  R103/RConn1 -- C103/LConn1
  C102/LConn1 -- R102/RConn1
  C101/LConn1 -- R101/RConn1
  SaturableReactor/LConn1 -- top/RConn1
  R303_replace/RConn1 -- R206/RConn1 -- Gto6/RConn1 -- C106/RConn1 -- bottom/RConn1
  R302_replace/LConn1 -- R203/LConn1 -- R103/LConn1 -- Gto2/RConn1 -- Gto3/LConn1 -- C102/RConn1 -- R202/RConn1 -- R301_replace/RConn1
  R206/LConn1 -- Gto5/RConn1 -- Gto6/LConn1 -- R106/LConn1 -- C105/RConn1 -- R205/RConn1
  R301_replace/LConn1 -- R101/LConn1 -- SaturableReactor/RConn1 -- Gto1/LConn1 -- R201/LConn1
  R104/LConn1 -- Gto3/RConn1 -- Gto4/LConn1 -- C103/RConn1 -- R203/RConn1 -- R204/LConn1
  R202/LConn1 -- R102/LConn1 -- C101/RConn1 -- Gto1/RConn1 -- Gto2/LConn1 -- R201/RConn1

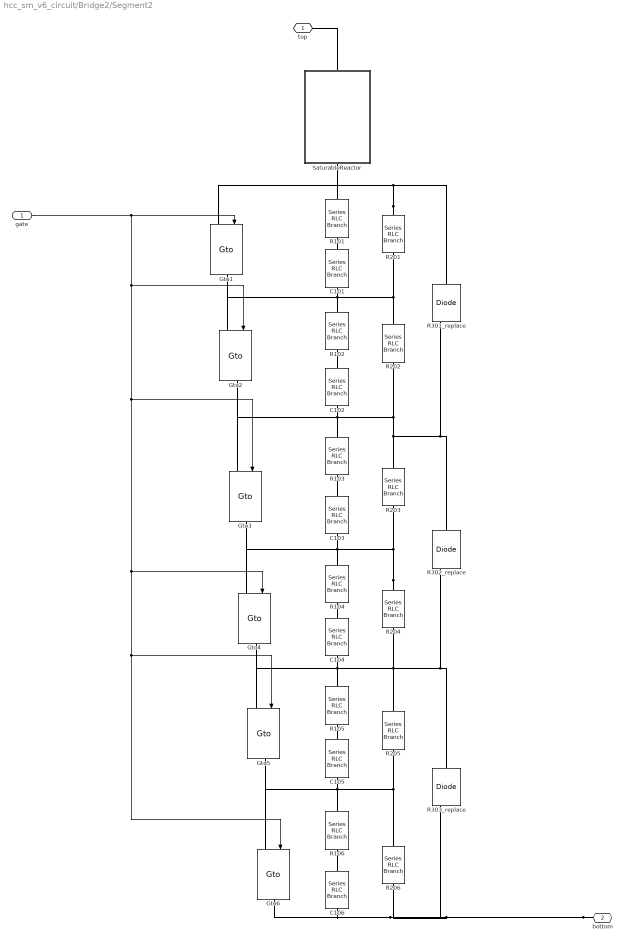
== system hcc_sm_v6_circuit/Bridge2/Segment2 ==
  gate : Inport
  C{101..106} (6 alike) : spsSeriesRLCBranchLib/Series RLC Branch  LConnTagsString=__new0  RConnTagsString=__new0  BranchType=C  Resistance=350  Inductance=107.42e-03  SetiL0=off  InitialCurrent=0  Capacitance=2.2*1e-6  Setx0=off  InitialVoltage=0  Measurements=None
  Gto{1..6} (6 alike) : spsGtoLib/Gto  Ron=0.226e-3  Lon=0  Vf=1.2  Tf=10e-6  Tt=20e-6  IC=0  Rs=161.25e3  Cs=0  Measurements=off
  R{101..106} (6 alike) : spsSeriesRLCBranchLib/Series RLC Branch  LConnTagsString=__new0  RConnTagsString=__new0  BranchType=R  Resistance=36  Inductance=107.42e-03  SetiL0=off  InitialCurrent=0  Capacitance=2.62e-06  Setx0=off  InitialVoltage=0  Measurements=None
  R{201..206} (6 alike) : spsSeriesRLCBranchLib/Series RLC Branch  LConnTagsString=__new0  RConnTagsString=__new0  BranchType=R  Resistance=88*1e3  Inductance=107.42e-03  SetiL0=off  InitialCurrent=0  Capacitance=2.62e-06  Setx0=off  InitialVoltage=0  Measurements=None
  R301_replace : spsDiodeLib/Diode  Ron=0.2624  Lon=0  Vf=11825.10104  IC=0  UseSnubber=0  Rs=1e6  Cs=0  Measurements=on
  R302_replace : spsDiodeLib/Diode  Ron=0.2624  Lon=0  Vf=11825.10104  IC=0  UseSnubber=0  Rs=1e6  Cs=0  Measurements=on
  R303_replace : spsDiodeLib/Diode  Ron=0.2624  Lon=0  Vf=11825.10104  IC=0  UseSnubber=0  Rs=1e6  Cs=0  Measurements=on
  SaturableReactor : Subsystem
  top : PMIOPort  Side=Left
  bottom : PMIOPort  Port=2  Side=Right
  wires:
  gate/1 -> Gto3/1, Gto4/1, Gto6/1, Gto5/1, Gto2/1, Gto1/1
  connections:
  R201/RConn1 -- Gto2/LConn1 -- Gto1/RConn1 -- C101/RConn1 -- R102/LConn1 -- R202/LConn1
  R204/LConn1 -- R203/RConn1 -- C103/RConn1 -- Gto4/LConn1 -- Gto3/RConn1 -- R104/LConn1
  R201/LConn1 -- Gto1/LConn1 -- SaturableReactor/RConn1 -- R101/LConn1 -- R301_replace/LConn1
  R205/RConn1 -- C105/RConn1 -- R106/LConn1 -- Gto6/LConn1 -- Gto5/RConn1 -- R206/LConn1
  R301_replace/RConn1 -- R202/RConn1 -- C102/RConn1 -- Gto3/LConn1 -- Gto2/RConn1 -- R103/LConn1 -- R203/LConn1 -- R302_replace/LConn1
  bottom/RConn1 -- C106/RConn1 -- Gto6/RConn1 -- R206/RConn1 -- R303_replace/RConn1
  SaturableReactor/LConn1 -- top/RConn1
  C101/LConn1 -- R101/RConn1
  C102/LConn1 -- R102/RConn1
  R103/RConn1 -- C103/LConn1
  R104/RConn1 -- C104/LConn1
  R105/RConn1 -- C105/LConn1
  R106/RConn1 -- C106/LConn1
  R302_replace/RConn1 -- R105/LConn1 -- C104/RConn1 -- Gto5/LConn1 -- Gto4/RConn1 -- R205/LConn1 -- R204/RConn1 -- R303_replace/LConn1

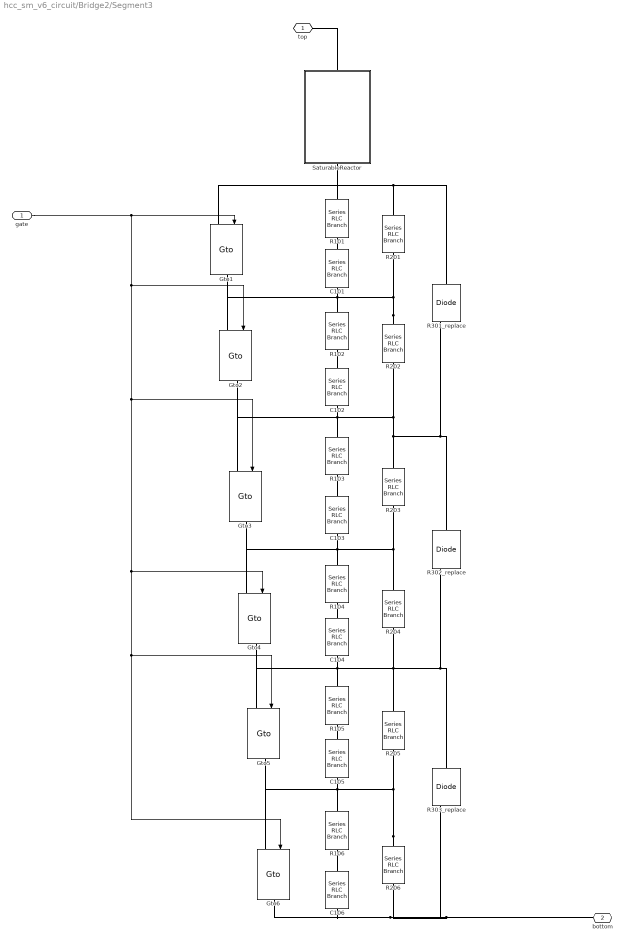
== system hcc_sm_v6_circuit/Bridge2/Segment3 ==
  gate : Inport
  C{101..106} (6 alike) : spsSeriesRLCBranchLib/Series RLC Branch  LConnTagsString=__new0  RConnTagsString=__new0  BranchType=C  Resistance=350  Inductance=107.42e-03  SetiL0=off  InitialCurrent=0  Capacitance=2.2*1e-6  Setx0=off  InitialVoltage=0  Measurements=None
  Gto{1..6} (6 alike) : spsGtoLib/Gto  Ron=0.226e-3  Lon=0  Vf=1.2  Tf=10e-6  Tt=20e-6  IC=0  Rs=161.25e3  Cs=0  Measurements=off
  R{101..106} (6 alike) : spsSeriesRLCBranchLib/Series RLC Branch  LConnTagsString=__new0  RConnTagsString=__new0  BranchType=R  Resistance=36  Inductance=107.42e-03  SetiL0=off  InitialCurrent=0  Capacitance=2.62e-06  Setx0=off  InitialVoltage=0  Measurements=None
  R{201..206} (6 alike) : spsSeriesRLCBranchLib/Series RLC Branch  LConnTagsString=__new0  RConnTagsString=__new0  BranchType=R  Resistance=88*1e3  Inductance=107.42e-03  SetiL0=off  InitialCurrent=0  Capacitance=2.62e-06  Setx0=off  InitialVoltage=0  Measurements=None
  R301_replace : spsDiodeLib/Diode  Ron=0.2624  Lon=0  Vf=11825.10104  IC=0  UseSnubber=0  Rs=1e6  Cs=0  Measurements=on
  R302_replace : spsDiodeLib/Diode  Ron=0.2624  Lon=0  Vf=11825.10104  IC=0  UseSnubber=0  Rs=1e6  Cs=0  Measurements=on
  R303_replace : spsDiodeLib/Diode  Ron=0.2624  Lon=0  Vf=11825.10104  IC=0  UseSnubber=0  Rs=1e6  Cs=0  Measurements=on
  SaturableReactor : Subsystem
  top : PMIOPort  Side=Left
  bottom : PMIOPort  Port=2  Side=Right
  wires:
  gate/1 -> Gto1/1, Gto2/1, Gto5/1, Gto6/1, Gto4/1, Gto3/1
  connections:
  R303_replace/LConn1 -- R204/RConn1 -- R205/LConn1 -- Gto4/RConn1 -- Gto5/LConn1 -- C104/RConn1 -- R105/LConn1 -- R302_replace/RConn1
  R106/RConn1 -- C106/LConn1
  R105/RConn1 -- C105/LConn1
  R104/RConn1 -- C104/LConn1
  R103/RConn1 -- C103/LConn1
  C102/LConn1 -- R102/RConn1
  C101/LConn1 -- R101/RConn1
  SaturableReactor/LConn1 -- top/RConn1
  R303_replace/RConn1 -- R206/RConn1 -- Gto6/RConn1 -- C106/RConn1 -- bottom/RConn1
  R302_replace/LConn1 -- R203/LConn1 -- R103/LConn1 -- Gto2/RConn1 -- Gto3/LConn1 -- C102/RConn1 -- R202/RConn1 -- R301_replace/RConn1
  R206/LConn1 -- Gto5/RConn1 -- Gto6/LConn1 -- R106/LConn1 -- C105/RConn1 -- R205/RConn1
  R301_replace/LConn1 -- R101/LConn1 -- SaturableReactor/RConn1 -- Gto1/LConn1 -- R201/LConn1
  R104/LConn1 -- Gto3/RConn1 -- Gto4/LConn1 -- C103/RConn1 -- R203/RConn1 -- R204/LConn1
  R202/LConn1 -- R102/LConn1 -- C101/RConn1 -- Gto1/RConn1 -- Gto2/LConn1 -- R201/RConn1

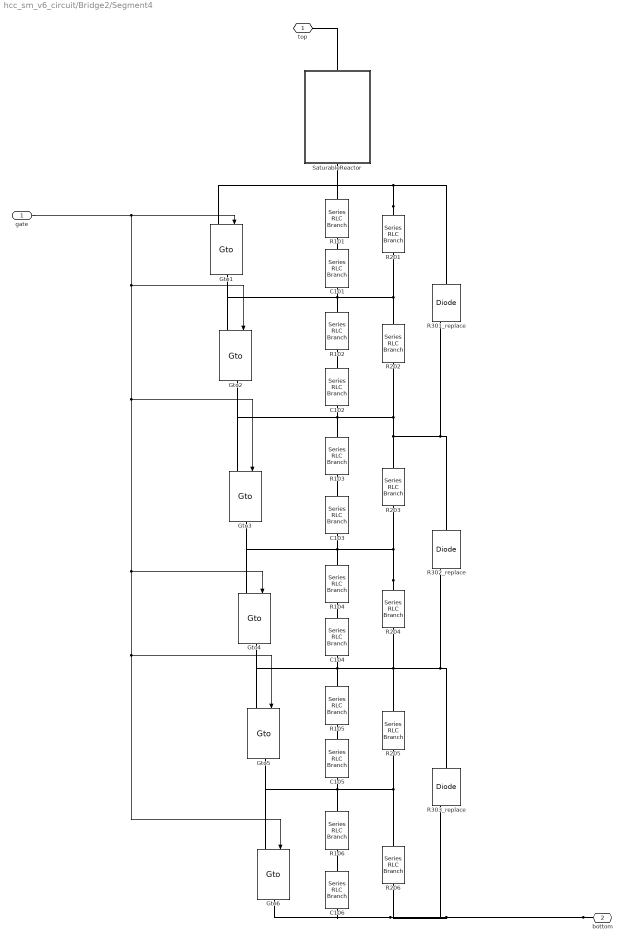
== system hcc_sm_v6_circuit/Bridge2/Segment4 ==
  gate : Inport
  C{101..106} (6 alike) : spsSeriesRLCBranchLib/Series RLC Branch  LConnTagsString=__new0  RConnTagsString=__new0  BranchType=C  Resistance=350  Inductance=107.42e-03  SetiL0=off  InitialCurrent=0  Capacitance=2.2*1e-6  Setx0=off  InitialVoltage=0  Measurements=None
  Gto{1..6} (6 alike) : spsGtoLib/Gto  Ron=0.226e-3  Lon=0  Vf=1.2  Tf=10e-6  Tt=20e-6  IC=0  Rs=161.25e3  Cs=0  Measurements=off
  R{101..106} (6 alike) : spsSeriesRLCBranchLib/Series RLC Branch  LConnTagsString=__new0  RConnTagsString=__new0  BranchType=R  Resistance=36  Inductance=107.42e-03  SetiL0=off  InitialCurrent=0  Capacitance=2.62e-06  Setx0=off  InitialVoltage=0  Measurements=None
  R{201..206} (6 alike) : spsSeriesRLCBranchLib/Series RLC Branch  LConnTagsString=__new0  RConnTagsString=__new0  BranchType=R  Resistance=88*1e3  Inductance=107.42e-03  SetiL0=off  InitialCurrent=0  Capacitance=2.62e-06  Setx0=off  InitialVoltage=0  Measurements=None
  R301_replace : spsDiodeLib/Diode  Ron=0.2624  Lon=0  Vf=11825.10104  IC=0  UseSnubber=0  Rs=1e6  Cs=0  Measurements=on
  R302_replace : spsDiodeLib/Diode  Ron=0.2624  Lon=0  Vf=11825.10104  IC=0  UseSnubber=0  Rs=1e6  Cs=0  Measurements=on
  R303_replace : spsDiodeLib/Diode  Ron=0.2624  Lon=0  Vf=11825.10104  IC=0  UseSnubber=0  Rs=1e6  Cs=0  Measurements=on
  SaturableReactor : Subsystem
  top : PMIOPort  Side=Left
  bottom : PMIOPort  Port=2  Side=Right
  wires:
  gate/1 -> Gto3/1, Gto4/1, Gto6/1, Gto5/1, Gto2/1, Gto1/1
  connections:
  R201/RConn1 -- Gto2/LConn1 -- Gto1/RConn1 -- C101/RConn1 -- R102/LConn1 -- R202/LConn1
  R204/LConn1 -- R203/RConn1 -- C103/RConn1 -- Gto4/LConn1 -- Gto3/RConn1 -- R104/LConn1
  R201/LConn1 -- Gto1/LConn1 -- SaturableReactor/RConn1 -- R101/LConn1 -- R301_replace/LConn1
  R205/RConn1 -- C105/RConn1 -- R106/LConn1 -- Gto6/LConn1 -- Gto5/RConn1 -- R206/LConn1
  R301_replace/RConn1 -- R202/RConn1 -- C102/RConn1 -- Gto3/LConn1 -- Gto2/RConn1 -- R103/LConn1 -- R203/LConn1 -- R302_replace/LConn1
  bottom/RConn1 -- C106/RConn1 -- Gto6/RConn1 -- R206/RConn1 -- R303_replace/RConn1
  SaturableReactor/LConn1 -- top/RConn1
  C101/LConn1 -- R101/RConn1
  C102/LConn1 -- R102/RConn1
  R103/RConn1 -- C103/LConn1
  R104/RConn1 -- C104/LConn1
  R105/RConn1 -- C105/LConn1
  R106/RConn1 -- C106/LConn1
  R302_replace/RConn1 -- R105/LConn1 -- C104/RConn1 -- Gto5/LConn1 -- Gto4/RConn1 -- R205/LConn1 -- R204/RConn1 -- R303_replace/LConn1

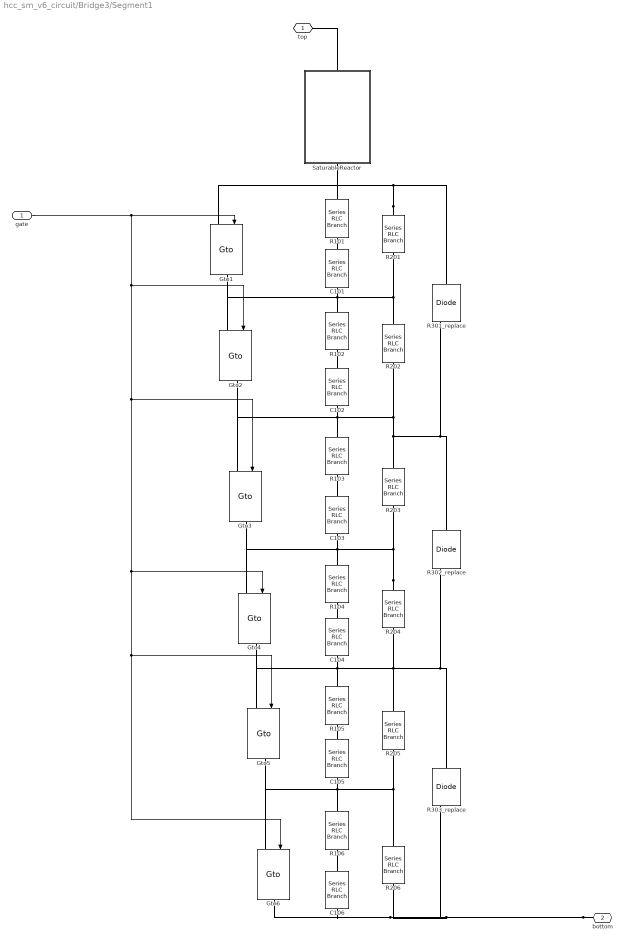
== system hcc_sm_v6_circuit/Bridge3/Segment1 ==
  gate : Inport
  C{101..106} (6 alike) : spsSeriesRLCBranchLib/Series RLC Branch  LConnTagsString=__new0  RConnTagsString=__new0  BranchType=C  Resistance=350  Inductance=107.42e-03  SetiL0=off  InitialCurrent=0  Capacitance=2.2*1e-6  Setx0=off  InitialVoltage=0  Measurements=None
  Gto{1..6} (6 alike) : spsGtoLib/Gto  Ron=0.226e-3  Lon=0  Vf=1.2  Tf=10e-6  Tt=20e-6  IC=0  Rs=161.25e3  Cs=0  Measurements=off
  R{101..106} (6 alike) : spsSeriesRLCBranchLib/Series RLC Branch  LConnTagsString=__new0  RConnTagsString=__new0  BranchType=R  Resistance=36  Inductance=107.42e-03  SetiL0=off  InitialCurrent=0  Capacitance=2.62e-06  Setx0=off  InitialVoltage=0  Measurements=None
  R{201..206} (6 alike) : spsSeriesRLCBranchLib/Series RLC Branch  LConnTagsString=__new0  RConnTagsString=__new0  BranchType=R  Resistance=88*1e3  Inductance=107.42e-03  SetiL0=off  InitialCurrent=0  Capacitance=2.62e-06  Setx0=off  InitialVoltage=0  Measurements=None
  R301_replace : spsDiodeLib/Diode  Ron=0.2624  Lon=0  Vf=11825.10104  IC=0  UseSnubber=0  Rs=1e6  Cs=0  Measurements=on
  R302_replace : spsDiodeLib/Diode  Ron=0.2624  Lon=0  Vf=11825.10104  IC=0  UseSnubber=0  Rs=1e6  Cs=0  Measurements=on
  R303_replace : spsDiodeLib/Diode  Ron=0.2624  Lon=0  Vf=11825.10104  IC=0  UseSnubber=0  Rs=1e6  Cs=0  Measurements=on
  SaturableReactor : Subsystem
  top : PMIOPort  Side=Left
  bottom : PMIOPort  Port=2  Side=Right
  wires:
  gate/1 -> Gto3/1, Gto4/1, Gto6/1, Gto5/1, Gto2/1, Gto1/1
  connections:
  R201/RConn1 -- Gto2/LConn1 -- Gto1/RConn1 -- C101/RConn1 -- R102/LConn1 -- R202/LConn1
  R204/LConn1 -- R203/RConn1 -- C103/RConn1 -- Gto4/LConn1 -- Gto3/RConn1 -- R104/LConn1
  R201/LConn1 -- Gto1/LConn1 -- SaturableReactor/RConn1 -- R101/LConn1 -- R301_replace/LConn1
  R205/RConn1 -- C105/RConn1 -- R106/LConn1 -- Gto6/LConn1 -- Gto5/RConn1 -- R206/LConn1
  R301_replace/RConn1 -- R202/RConn1 -- C102/RConn1 -- Gto3/LConn1 -- Gto2/RConn1 -- R103/LConn1 -- R203/LConn1 -- R302_replace/LConn1
  bottom/RConn1 -- C106/RConn1 -- Gto6/RConn1 -- R206/RConn1 -- R303_replace/RConn1
  SaturableReactor/LConn1 -- top/RConn1
  C101/LConn1 -- R101/RConn1
  C102/LConn1 -- R102/RConn1
  R103/RConn1 -- C103/LConn1
  R104/RConn1 -- C104/LConn1
  R105/RConn1 -- C105/LConn1
  R106/RConn1 -- C106/LConn1
  R302_replace/RConn1 -- R105/LConn1 -- C104/RConn1 -- Gto5/LConn1 -- Gto4/RConn1 -- R205/LConn1 -- R204/RConn1 -- R303_replace/LConn1
